simulink subsystem "Bluetooth_Total"  (R2024b)
settings: Solver=VariableStepAuto  StartTime=0.0  StopTime=10.0  RelTol=1e-3
settings Model: Creator=Chenfu  LastModifiedBy=Chenfu

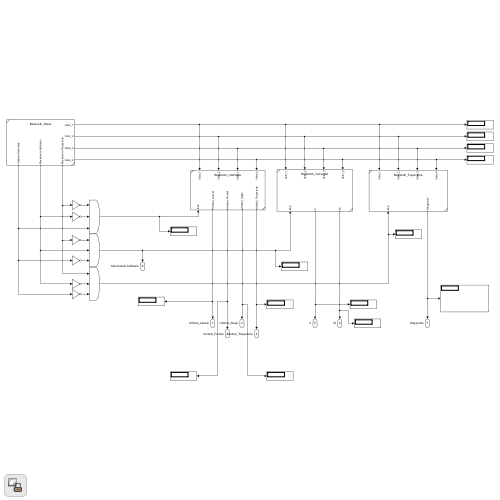
[thumbnail: Simulink's stored preview of the top-level diagram]
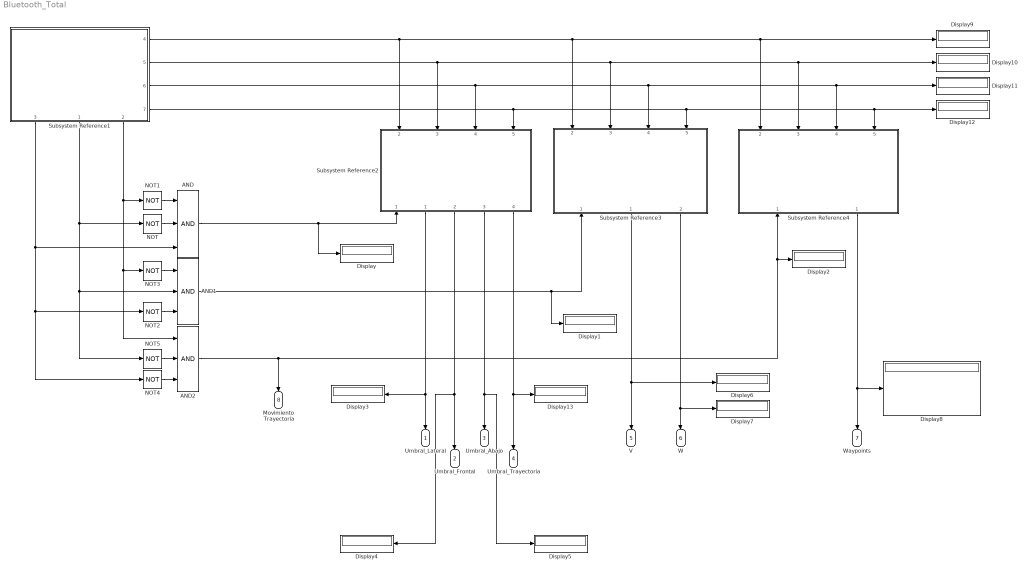
== system Bluetooth_Total ==
  AND : Logic  Inputs=3  IconShape=distinctive  AllPortsSameDT=off  OutDataTypeStr=boolean
  AND1 : Logic  Inputs=3  IconShape=distinctive  AllPortsSameDT=off  OutDataTypeStr=boolean
  AND2 : Logic  Inputs=3  IconShape=distinctive  AllPortsSameDT=off  OutDataTypeStr=boolean
  Display{,1..13} (14 alike) : Display
  NOT{,1..5} (6 alike) : Logic  Operator=NOT  IconShape=distinctive  AllPortsSameDT=off  OutDataTypeStr=boolean
  Subsystem Reference1 : Subsystem  ReferencedSubsystem=Bluetooth_Datos
      settings: PortSchema="{\"entries\":[{\"content\":{\"sides\":[{\"content\":{},\"type\":\"ConnectorPlacement.EquallySpacedRectSide\",\"uuid\":\"85e48fc4-7fef-4e3a-b6b7-544efc632718\"},{\"content\":{\"connectorIds\":[\"Out4\",\"Out5\",\"Out6\",\"Out7\"],\"side\":\"RIGHT\"},\"type\":\"ConnectorPlacement.EquallySpacedRectSide\",\"uuid\":\"dc8dcd29-daa3-4d51-ad95-5b30a08c4b18\"},{\"content\":{\"side\":\"TOP\"},\"type\":\"ConnectorPlacement.EquallySpacedRectSide\",\"uuid\":\"90e8e681-e3a3-45f3-b97e-b02ee187e4d2\"},{\"content\":{\"connectorIds\":[\"Out3\",\"Out1\",\"Out2\"],\"side\":\"BOTTOM\"},\"type\":\"ConnectorPlacement.EquallySpacedRectSide\",\"uuid\":\"80684380-6c99-4e98-b9b8-2fb3496b12c7\"}]},\"type\":\"ConnectorPlacement.EquallySpacedConnector\",\"uuid\":\"e547c7f5-4d5c-4219-925b-a3e1854c8f15\"}],\"packageUris\":[\"http://schema.mathworks.com/mf0/Connector/R2020b\"],\"version\":\"1.0\"}"
  Subsystem Reference2 : Subsystem  ReferencedSubsystem=Bluetooth_Umbrales
      settings: PortSchema="{\"entries\":[{\"content\":{\"sides\":[{\"content\":{},\"type\":\"ConnectorPlacement.EquallySpacedRectSide\",\"uuid\":\"6fa65170-c700-46c9-8b43-e8886770a893\"},{\"content\":{\"side\":\"RIGHT\"},\"type\":\"ConnectorPlacement.EquallySpacedRectSide\",\"uuid\":\"5046e329-eec3-4b21-a258-65bfd46f7856\"},{\"content\":{\"connectorIds\":[\"In2\",\"In3\",\"In4\",\"In5\"],\"side\":\"TOP\"},\"type\":\"ConnectorPlacement.EquallySpacedRectSide\",\"uuid\":\"b17b81e4-943e-4aa5-af29-29ab5a99f1ef\"},{\"content\":{\"connectorIds\":[\"In1\",\"Out1\",\"Out2\",\"Out3\",\"Out4\"],\"side\":\"BOTTOM\"},\"type\":\"ConnectorPlacement.EquallySpacedRectSide\",\"uuid\":\"16e00616-1ef0-4943-88f1-44ad50b2407a\"}]},\"type\":\"ConnectorPlacement.EquallySpacedConnector\",\"uuid\":\"f253d6c0-32c9-4dcd-9004-eb58c19c4f9b\"}],\"packageUris\":[\"http://schema.mathworks.com/mf0/Connector/R2020b\"],\"version\":\"1.0\"}"
  Subsystem Reference3 : Subsystem  ReferencedSubsystem=Bluetooth_Velocidad
      settings: PortSchema="{\"entries\":[{\"content\":{\"sides\":[{\"content\":{},\"type\":\"ConnectorPlacement.EquallySpacedRectSide\",\"uuid\":\"351abf9b-a583-4037-afe6-de49ebd5a9e5\"},{\"content\":{\"side\":\"RIGHT\"},\"type\":\"ConnectorPlacement.EquallySpacedRectSide\",\"uuid\":\"344b1dd7-6b36-4189-9b21-7e3fabac2519\"},{\"content\":{\"connectorIds\":[\"In2\",\"In3\",\"In4\",\"In5\"],\"side\":\"TOP\"},\"type\":\"ConnectorPlacement.EquallySpacedRectSide\",\"uuid\":\"391aa8ea-a515-421b-9ff4-f213cec3ce89\"},{\"content\":{\"connectorIds\":[\"In1\",\"Out1\",\"Out2\"],\"side\":\"BOTTOM\"},\"type\":\"ConnectorPlacement.EquallySpacedRectSide\",\"uuid\":\"ac7317b7-9d7b-4274-96fe-8769e9539390\"}]},\"type\":\"ConnectorPlacement.EquallySpacedConnector\",\"uuid\":\"66339ee2-3d48-4931-9bdf-949e45aca2cd\"}],\"packageUris\":[\"http://schema.mathworks.com/mf0/Connector/R2020b\"],\"version\":\"1.0\"}"
  Subsystem Reference4 : Subsystem  ReferencedSubsystem=Bluetooth_Trayectoria
      settings: PortSchema="{\"entries\":[{\"content\":{\"sides\":[{\"content\":{},\"type\":\"ConnectorPlacement.EquallySpacedRectSide\",\"uuid\":\"fa3df764-8cb1-47b4-9f16-ffb2b486d14a\"},{\"content\":{\"side\":\"RIGHT\"},\"type\":\"ConnectorPlacement.EquallySpacedRectSide\",\"uuid\":\"a0b0ca70-930b-4ef5-81d4-646f3164df97\"},{\"content\":{\"connectorIds\":[\"In2\",\"In3\",\"In4\",\"In5\"],\"side\":\"TOP\"},\"type\":\"ConnectorPlacement.EquallySpacedRectSide\",\"uuid\":\"f01310ed-7edf-4a5a-b003-59e7f50ba3e0\"},{\"content\":{\"connectorIds\":[\"In1\",\"Out1\"],\"side\":\"BOTTOM\"},\"type\":\"ConnectorPlacement.EquallySpacedRectSide\",\"uuid\":\"96c356d0-ac0d-415f-b60c-662a0d1805ac\"}]},\"type\":\"ConnectorPlacement.EquallySpacedConnector\",\"uuid\":\"0436bb49-f68b-4eed-81e1-e5385678400e\"}],\"packageUris\":[\"http://schema.mathworks.com/mf0/Connector/R2020b\"],\"version\":\"1.0\"}"
  Umbral_Lateral : Outport  OutDataTypeStr=double
  Umbral_Frontal : Outport  Port=2  OutDataTypeStr=double
  Umbral_Abajo : Outport  Port=3  OutDataTypeStr=double
  Umbral_Trayectoria : Outport  Port=4  OutDataTypeStr=double
  V : Outport  Port=5  OutDataTypeStr=double
  W : Outport  Port=6  OutDataTypeStr=double
  Waypoints : Outport  Port=7  OutDataTypeStr=double
  Movimiento Trayectoria : Outport  Port=8
  wires:
  NOT3/1 -> AND1/1
  AND1/1 -> Subsystem Reference3/1, Display1/1
  Subsystem Reference1/7 -> Subsystem Reference2/5, Subsystem Reference4/5, Display12/1, Subsystem Reference3/5
  NOT5/1 -> AND2/2
  Subsystem Reference1/1 -> NOT5/1, AND1/2, NOT/1
  Subsystem Reference1/3 -> NOT4/1, NOT2/1, AND/3
  Subsystem Reference1/5 -> Subsystem Reference3/3, Display10/1, Subsystem Reference4/3, Subsystem Reference2/3
  NOT4/1 -> AND2/3
  Subsystem Reference1/4 -> Display9/1, Subsystem Reference4/2, Subsystem Reference3/2, Subsystem Reference2/2
  Subsystem Reference1/2 -> AND2/1, NOT3/1, NOT1/1
  AND/1 -> Display/1, Subsystem Reference2/1
  AND2/1 -> Subsystem Reference4/1, Display2/1, Movimiento Trayectoria/1
  NOT2/1 -> AND1/3
  NOT/1 -> AND/2
  Subsystem Reference1/6 -> Display11/1, Subsystem Reference4/4, Subsystem Reference3/4, Subsystem Reference2/4
  NOT1/1 -> AND/1
  Subsystem Reference2/1 -> Umbral_Lateral/1, Display3/1
  Subsystem Reference2/2 -> Display4/1, Umbral_Frontal/1
  Subsystem Reference4/1 -> Display8/1, Waypoints/1
  Subsystem Reference3/2 -> Display7/1, W/1
  Subsystem Reference3/1 -> Display6/1, V/1
  Subsystem Reference2/3 -> Display5/1, Umbral_Abajo/1
  Subsystem Reference2/4 -> Display13/1, Umbral_Trayectoria/1
